simulink model "Bo_KDXCS_dieu_khien_DC_1c"  (R2019a)
settings: Solver=VariableStepAuto  StartTime=0.0  StopTime=10  RelTol=1e-3
libraries: powerlib x8
settings Model: Creator=Admin  LastModifiedBy=Admin

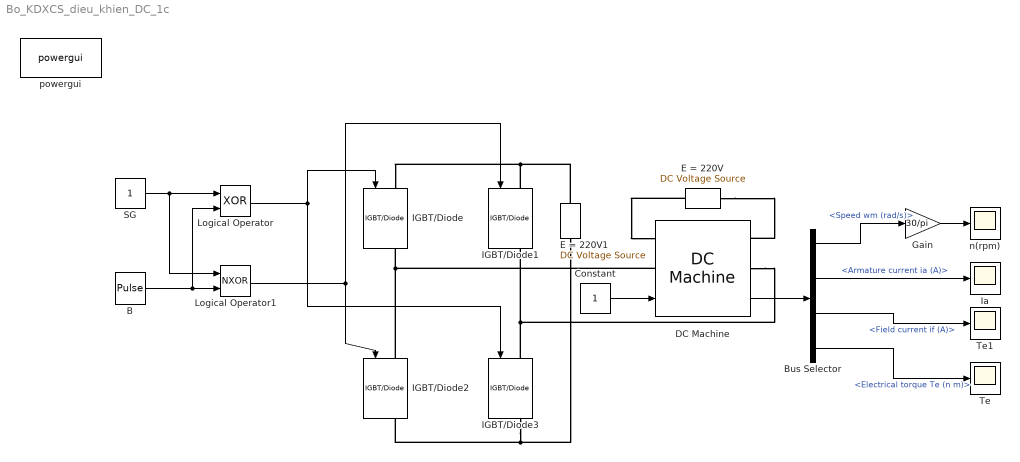
== system Bo_KDXCS_dieu_khien_DC_1c ==
  B : DiscretePulseGenerator  PulseType=Time based  Period=0.02  PulseWidth=50
  Bus Selector : BusSelector  OutputSignals=Speed wm (rad/s),Armature current ia (A),Field current if (A),Electrical torque Te (n m)
  Constant : Constant
  DC Machine : powerlib/Machines/DC Machine  PresetModel=No  MechanicalLoad=Torque TL  FieldType=Wound  ShowDetailedParameters=on  MeasurementBus=off  RLa=[0.2305 0.023]  RLf=[298 59.6]  Laf=1.247  MachineConstant=Torque constant (N.m/A)  Ke=1.8  Kt=1.8  J=0.28  Bm=1.58e-4  Tf=1.75  w0=1  Ifinit=1  TsPowergui=0  TsBlock=-1
  E = 220V : powerlib/Electrical Sources/DC Voltage Source  Amplitude=220  Measurements=None
  E = 220V1 : powerlib/Electrical Sources/DC Voltage Source  Amplitude=220  Measurements=None
  Gain : Gain  Gain=30/pi
  IGBT/Diode{,1..3} (4 alike) : powerlib/Power Electronics/IGBT//Diode  Ron=1e-3  Rs=1e5  Cs=inf  Measurements=on
      settings: SourceProductName=Simscape Electrical
  "Ia " : Scope
  Logical Operator : Logic  Operator=XOR  AllPortsSameDT=off  OutDataTypeStr=boolean
  Logical Operator1 : Logic  Operator=NXOR  AllPortsSameDT=off  OutDataTypeStr=boolean
  "SG " : Constant
  Te : Scope
  Te1 : Scope
  "n(rpm) " : Scope
  powergui : powerlib/powergui  Priority=1  SimulationMode=Continuous  SampleTime=50e-6  frequency=60  Iterations=50  frequencyindice=0  Pbase=100e6  ErrMax=1e-4  UnitsV=kV  UnitsW=MW  buscounter=0  FunctionMessages=off  echomessages=off  EnableUseOfTLC=off  CurrentSourceSwitches=off  DisableSnubberDevices=off  DisableRonSwitches=off  DisableVfSwitches=off  DisplayEquations=off  AutomaticDiscreteSolvers=off  SolverType=Tustin/Backward Euler (TBE)  Interpol=off  ExternalGateDelay=off  methode=off  Ts=100  x0status=blocks  SPID=on  SwTol=0  HookPort=off  NonlinearTolerance=0  nMaxIteration=15  ContinueOnMaxIteration=off  RestoreLinks=warning  ResistiveCurrentMeasurement=off  Frange=[0:2:500]  Ylog=off  Xlog=on  ShowGrid=off  save=off  variable=ZData  structure=0  ZoomFFT=off  StartTime=0.0  cycles=1  DisplayStyle=1  fundamental=60  FreqAxis=off  MaxFrequency=1000  frequencyindicesteady=1  RmsSteady=1  display=off
      settings: SourceProductName=Simscape Electrical
  wires:
  Constant/1 -> DC Machine/1
  Logical Operator1/1 -> IGBT/Diode2/1, IGBT/Diode1/1
  Logical Operator/1 -> IGBT/Diode3/1, IGBT/Diode/1
  Gain/1 -> "n(rpm) "/1
  Bus Selector/3 -> Te1/1  "<Field current if (A)>"
  Bus Selector/2 -> "Ia "/1  "<Armature current ia (A)>"
  Bus Selector/4 -> Te/1  "<Electrical torque Te (n m)>"
  Bus Selector/1 -> Gain/1  "<Speed wm (rad/s)>"
  DC Machine/1 -> Bus Selector/1
  "SG "/1 -> Logical Operator1/1, Logical Operator/1
  B/1 -> Logical Operator/2, Logical Operator1/2
  connections:
  IGBT/Diode2/LConn1 -- IGBT/Diode/RConn1 -- DC Machine/LConn1
  IGBT/Diode3/LConn1 -- IGBT/Diode1/RConn1 -- DC Machine/RConn1
  E = 220V/LConn1 -- DC Machine/RConn2
  E = 220V/RConn1 -- DC Machine/LConn2
  E = 220V1/RConn1 -- IGBT/Diode1/LConn1 -- IGBT/Diode/LConn1
  E = 220V1/LConn1 -- IGBT/Diode3/RConn1 -- IGBT/Diode2/RConn1
